simulink model "AION_auto_mode_request"  (R2021a)
settings: configuration reference "AION_IDS_Speedgoat" (kept outside this file)
undefined symbols (not defined in the file): set_ADCU_info
settings Model: DataDictionary=AION_auto_mode_request.sldd  SimulationMode=external  Creator=Administrator  LastModifiedBy=Administrator
settings ConfigSetRef: SourceName=AION_IDS_Speedgoat

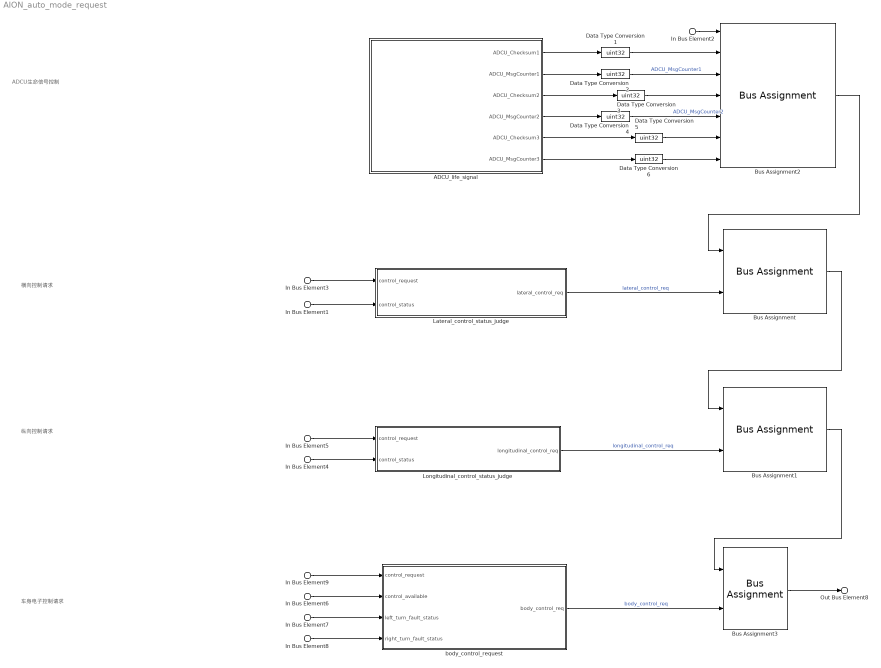
== system AION_auto_mode_request ==
  note: ADCU生命信号控制
  note: 横向控制请求
  note: 纵向控制请求
  note: 车身电子控制请求
  In Bus Element2 : Inport  PortName=InBus
  In Bus Element3 : Inport  PortName=InBus  Element=set_lateral_control_info.set_LatCtrlReq
  In Bus Element5 : Inport  PortName=InBus  Element=set_longitudinal_control_info.set_LngCtrlReq
  In Bus Element9 : Inport  PortName=InBus  Element=set_ADCU_info.set_BodyCtrlReq
  In Bus Element1 : Inport  PortName=InBus  Element=get_SCU_info.get_LatCtrlMode
  In Bus Element4 : Inport  PortName=InBus  Element=get_SCU_info.get_LngCtrlMode
  In Bus Element6 : Inport  PortName=InBus  Element=get_BCM_info.get_CtrlAvailable
  In Bus Element7 : Inport  PortName=InBus  Element=get_BCM_info.get_LeftTurnLampFaultSt
  In Bus Element8 : Inport  PortName=InBus  Element=get_BCM_info.get_RightTurnLampFaultSt
  ADCU_life_signal : MATLAB Function  TreatAsAtomicUnit=on
  Bus Assignment : BusAssignment  AssignedSignals=set_lateral_control_info.set_LatCtrlReq
  Bus Assignment1 : BusAssignment  AssignedSignals=set_longitudinal_control_info.set_LngCtrlReq
  Bus Assignment2 : BusAssignment  AssignedSignals=set_ADCU_info.set_Checksum1,set_ADCU_info.set_MsgCounter1,set_ADCU_info.set_Checksum2,set_ADCU_info.set_MsgCounter2,set_ADCU_info.set_Checksum3,set_ADCU_info.set_MsgCounter3
  Bus Assignment3 : BusAssignment  AssignedSignals=set_ADCU_info.set_BodyCtrlReq
  Data Type Conversion{1..6} (6 alike) : DataTypeConversion  OutDataTypeStr=uint32
  Lateral_control_status_judge : MATLAB Function  TreatAsAtomicUnit=on
  Longitudinal_control_status_judge : MATLAB Function  TreatAsAtomicUnit=on
  body_control_request : MATLAB Function  TreatAsAtomicUnit=on
  Out Bus Element8 : Outport  PortName=OutBus
  wires:
  Lateral_control_status_judge/1(lateral_control_req) -> Bus Assignment/2  "lateral_control_req"
  In Bus Element2/1 -> Bus Assignment2/1
  Bus Assignment/1 -> Bus Assignment1/1
  In Bus Element4/1 -> Longitudinal_control_status_judge/2(control_status)
  Longitudinal_control_status_judge/1(longitudinal_control_req) -> Bus Assignment1/2  "longitudinal_control_req"
  In Bus Element3/1 -> Lateral_control_status_judge/1(control_request)
  In Bus Element5/1 -> Longitudinal_control_status_judge/1(control_request)
  In Bus Element1/1 -> Lateral_control_status_judge/2(control_status)
  Bus Assignment2/1 -> Bus Assignment/1
  ADCU_life_signal/2(ADCU_MsgCounter1) -> Data Type Conversion2/1
  ADCU_life_signal/4(ADCU_MsgCounter2) -> Data Type Conversion4/1
  ADCU_life_signal/6(ADCU_MsgCounter3) -> Data Type Conversion6/1
  ADCU_life_signal/1(ADCU_Checksum1) -> Data Type Conversion1/1
  ADCU_life_signal/3(ADCU_Checksum2) -> Data Type Conversion3/1
  ADCU_life_signal/5(ADCU_Checksum3) -> Data Type Conversion5/1
  Data Type Conversion1/1 -> Bus Assignment2/2
  Data Type Conversion2/1 -> Bus Assignment2/3  "ADCU_MsgCounter1"
  Data Type Conversion3/1 -> Bus Assignment2/4
  Data Type Conversion4/1 -> Bus Assignment2/5  "ADCU_MsgCounter2"
  Data Type Conversion5/1 -> Bus Assignment2/6
  Data Type Conversion6/1 -> Bus Assignment2/7
  In Bus Element6/1 -> body_control_request/2(control_available)
  In Bus Element9/1 -> body_control_request/1(control_request)
  In Bus Element7/1 -> body_control_request/3(left_turn_fault_status)
  In Bus Element8/1 -> body_control_request/4(right_turn_fault_status)
  Bus Assignment1/1 -> Bus Assignment3/1
  Bus Assignment3/1 -> Out Bus Element8/1
  body_control_request/1(body_control_req) -> Bus Assignment3/2  "body_control_req"

== matlab function AION_auto_mode_request/Longitudinal_control_status_judge ==
  data: control_request input; control_status input Enum: Control_status size=1; longitudinal_control_req output Enum: Control_request size=1
% 操作模式判断
function longitudinal_control_req = longitudinal_control_status_judge(control_request,control_status)
%   1.输入参数：
%       (1)control_request           纵向控制请求的实际值
%       (2)control_status            纵向控制功能状态
        
%   2.输出参数：
%       (1)longitudinal_control_req       纵向控制请求的期望值

%%
if(control_request == Control_request.Auto)
    %车辆上电过程，使车辆进入自动控制状态
    switch control_status 
        case Control_status.QuitStatus
        longitudinal_control_req = Control_request.Manual;
        case Control_status.ManualStatus
        longitudinal_control_req = Control_request.Auto;
         case Control_status.AutoStatus
        longitudinal_control_req = Control_request.Auto;
        otherwise
        longitudinal_control_req = Control_request.Manual;
    end
else
    longitudinal_control_req = Control_request.Manual;
end
end

== matlab function AION_auto_mode_request/Lateral_control_status_judge ==
  data: control_request input; control_status input Enum: Control_status size=1; lateral_control_req output Enum: Control_request size=1
% 操作模式判断
function lateral_control_req = lateral_control_status_judge(control_request,control_status)
%   1.输入参数：
%       (1)control_status            横向控制功能状态
%   2.输出参数：
%       (1)lateral_control_req       横向控制请求

%%

if(control_request == Control_request.Auto)
%     车辆上电过程，使车辆进入自动控制状态
    switch control_status 
        case Control_status.QuitStatus
        lateral_control_req = Control_request.Manual;
        case Control_status.ManualStatus
        lateral_control_req = Control_request.Auto;
        case Control_status.AutoStatus
        lateral_control_req = Control_request.Auto;
        otherwise %Fault_status
        lateral_control_req = Control_request.Manual;
    end
else
    lateral_control_req = Control_request.Manual;
end

% lateral_control_req = Control_request.Manual;
end

== matlab function AION_auto_mode_request/ADCU_life_signal ==
  data: ADCU_Checksum1 output; ADCU_MsgCounter1 output; ADCU_Checksum2 output; ADCU_MsgCounter2 output; ADCU_Checksum3 output; ADCU_MsgCounter3 output
function [ADCU_Checksum1,ADCU_MsgCounter1,ADCU_Checksum2,ADCU_MsgCounter2,ADCU_Checksum3,ADCU_MsgCounter3] = ADCU_life_signal()

%% 静态变量声明及初始化
% 初始化
persistent adcu_msg_count
if isempty(adcu_msg_count)
   adcu_msg_count = 0;
end

%% 计算checksum
% msgcounter在0-15之间循环变化
if(adcu_msg_count > 15)
    adcu_msg_count = 0;
end
ADCU_MsgCounter1 = adcu_msg_count;
ADCU_MsgCounter2 = adcu_msg_count;
ADCU_MsgCounter3 = adcu_msg_count;
adcu_msg_count = adcu_msg_count + 1;

ADCU_Checksum1 = 1;
ADCU_Checksum2 = 1;
ADCU_Checksum3 = 1;

end

== matlab function AION_auto_mode_request/body_control_request ==
  data: control_request input; body_control_req output; control_available input; left_turn_fault_status input; right_turn_fault_status input
function body_control_req = body_control_status(control_request,control_available,left_turn_fault_status,right_turn_fault_status)

%%
%ADCU 确认 BCM_CtrlAvailable = Available；
%ADCU 确认转向灯 没有故障 ， 即 BCM_LeftTurnLampFaultSt = Not Fault && BCM_RightTurnLampFaultSt = Not Fault；

if(control_request == Enable_request.Enable)
    if((control_available == Available_status.Available)&&(left_turn_fault_status == Fault_status.NotFault)&&(right_turn_fault_status == Fault_status.NotFault))
          body_control_req = Enable_request.Enable;     
    else
      body_control_req = Enable_request.Disable;
    end
else
    body_control_req = Enable_request.Disable;
end

end
